simulink model "dinamica_estabilidad2017b"  (R2017b)
settings: Solver=ode23  StartTime=0.0  StopTime=20  RelTol=1e-3
libraries: eeGeneralControl x1, simulink x1
settings Model: Creator=raulD
settings DataIOCC: ReturnWorkspaceOutputs=on
settings DebuggingCC: UnconnectedInputMsg=none  UnconnectedOutputMsg=none  UnconnectedLineMsg=none
settings ModelReferenceCC: EnableRefExpFcnMdlSchedulingChecks=off
settings SFSimCC: SimUseLocalCustomCode=on
settings RTWCC: Description=Generic Real-Time Target  RTWUseLocalCustomCode=on

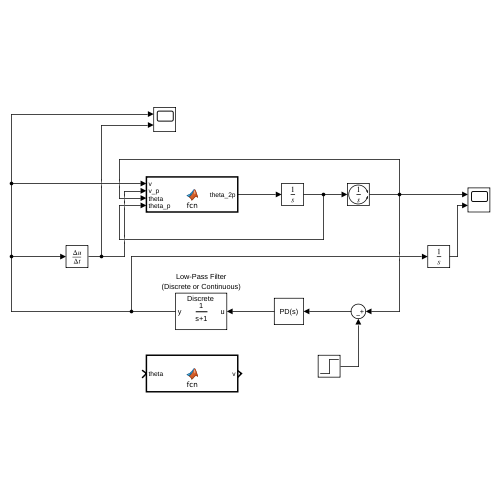
[thumbnail: Simulink's stored preview of the top-level diagram]
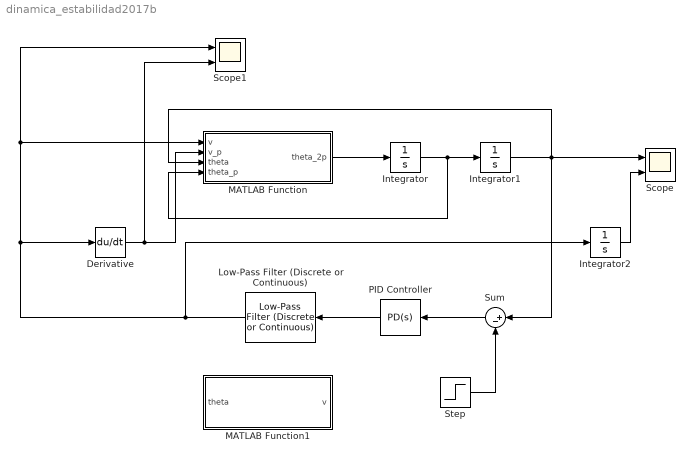
== system dinamica_estabilidad2017b ==
  Derivative : Derivative
  Integrator : Integrator
  Integrator1 : Integrator  WrapState=on  WrappedStateUpperValue=2*pi  WrappedStateLowerValue=0
  Integrator2 : Integrator
  Low-Pass Filter (Discrete or Continuous) : eeGeneralControl/Low-Pass Filter (Discrete or Continuous)  K=1  T=1  B=inf  A=-inf  init_option=Inherited from block input  x0=0  Ts=-1
  MATLAB Function : MATLAB Function  TreatAsAtomicUnit=on
  MATLAB Function1 : MATLAB Function  TreatAsAtomicUnit=on
  PID Controller : simulink/Continuous/PID Controller  Controller=PD  Form=Parallel  TimeDomain=Continuous-time  SampleTime=-1  IntegratorMethod=Forward Euler  ControllerParametersSource=internal  P=1  I=1  D=0.01  N=10  UseFilter=on  TunerSelectOption=Transfer Function Based (PID Tuner App)  InitialConditionSource=internal  InitialConditionForIntegrator=0  InitialConditionForFilter=0  DifferentiatorICPrevScaledInput=0  ExternalReset=none  TrackingMode=off  Kt=1  LimitOutput=off  UpperSaturationLimit=inf  LowerSaturationLimit=-inf  LinearizeAsGain=on  AntiWindupMode=none  Kb=1  POutMin=[]  POutMax=[]  IOutMin=[]  IOutMax=[]  DOutMin=[]  DOutMax=[]  NOutMin=[]  NOutMax=[]  SumOutMin=[]  SumOutMax=[]  SaturationOutMin=[]  SaturationOutMax=[]  PParamMin=[]  PParamMax=[]  IParamMin=[]  IParamMax=[]  DParamMin=[]  DParamMax=[]  NParamMin=[]  NParamMax=[]  KbParamMin=[]  KbParamMax=[]  KtParamMin=[]  KtParamMax=[]  KbOutMin=[]  KbOutMax=[]  KtOutMin=[]  KtOutMax=[]  IntegratorOutMin=[]  IntegratorOutMax=[]  FilterOutMin=[]  FilterOutMax=[]  SumI1OutMin=[]  SumI1OutMax=[]  SumI2OutMin=[]  SumI2OutMax=[]  SumI3OutMin=[]  SumI3OutMax=[]  SumDOutMin=[]  SumDOutMax=[]  DifferentiatorOutMin=[]  DifferentiatorOutMax=[]  FilterDiffOutCoefMin=[]  FilterDiffOutCoefMax=[]  ReciprocalOutMin=[]  ReciprocalOutMax=[]  SumDenOutMin=[]  SumDenOutMax=[]  SumNumOutMin=[]  SumNumOutMax=[]  DivideOutMin=[]  DivideOutMax=[]  IntegratorContinuousStateAttributes=''  IntegratorStateMustResolveToSignalObject=off  IntegratorRTWStateStorageClass=Auto  FilterContinuousStateAttributes=''  FilterStateMustResolveToSignalObject=off  FilterRTWStateStorageClass=Auto  InitialConditionSetting=State (most efficient)
  Scope : Scope  NumInputPorts=2
  Scope1 : Scope  NumInputPorts=2
  Step : Step  After=1*pi/180  SampleTime=0
  Sum : Sum  Inputs=|+-
  wires:
  MATLAB Function/1(theta_2p) -> Integrator/1
  Integrator/1 -> Integrator1/1, MATLAB Function/4(theta_p)
  Integrator1/1 -> Sum/1, MATLAB Function/3(theta), Scope/1
  Derivative/1 -> Scope1/2, MATLAB Function/2(v_p)
  Integrator2/1 -> Scope/2
  PID Controller/1 -> Low-Pass Filter (Discrete or Continuous)/1
  Sum/1 -> PID Controller/1
  Step/1 -> Sum/2
  Low-Pass Filter (Discrete or Continuous)/1 -> Integrator2/1, Derivative/1, Scope1/1, MATLAB Function/1(v)

== matlab function dinamica_estabilidad2017b/MATLAB Function1 ==
  data: v output; theta input
function v = fcn(theta)

g = 9.8;
L = 20e-2;
beta_v = 0.2;
M = 40e-2;
m = 1;

Ts = 1/100;
k = -2*beta_v*cos(theta)/(L*(-m*cos(theta)+M+m));

x_k1_1 = 1*x_k_1 + Ts*x_k_2;
x_k1_2 = 1*x_k_2 + Ts*x_k_3;
x_k1_3 = 1*x_k_3;

kd = 1;
kp = 10;
v = 1/k*(-x_k1_3-kd*x_k1_2-kp*x_k1_1);

== matlab function dinamica_estabilidad2017b/MATLAB Function ==
  data: theta_2p output; v input; v_p input; theta input; theta_p input
function theta_2p = fcn(v, v_p, theta, theta_p)

g = 9.8;
L = 20e-2;
beta_v = 0.2;
M = 40e-2;
m = 1;

theta_2p = (g*m*sin(theta) - m*v_p*cos(theta) - 2*beta_v*v*cos(theta) + m*v_p*cos(theta)^3 + m*cos(theta)^2*sin(theta) - M*v_p*cos(theta) + M*g*sin(theta) + 2*L*m*theta_p^2*cos(theta)*sin(theta))/(L*(- m*cos(theta)^2 + M + m));
